simulink subsystem "ForwardDynamics"  (R2022a)
settings: Solver=VariableStepAuto  StartTime=0.0  StopTime=10.0  RelTol=1e-3
model mask{spaceRobot=SpaceRobot, SimulateUsing=Code generation}
  mask prompts: SimulateUsing "SystemBlock:MATLABSystem:SimulateUsing"
settings Model: Creator=charl  LastModifiedBy=charl

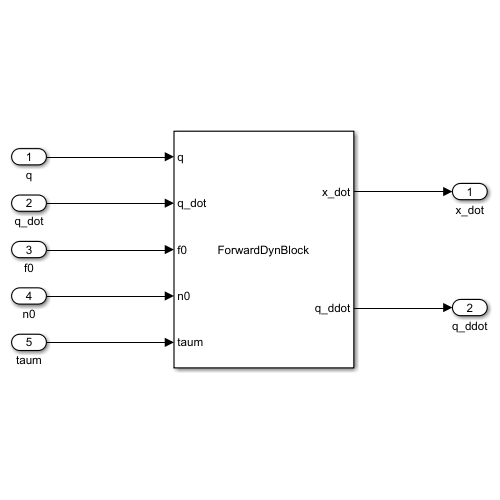
[thumbnail: Simulink's stored preview of the top-level diagram]
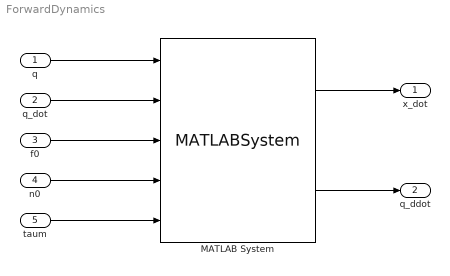
== system ForwardDynamics ==
  q : Inport
  q_dot : Inport  Port=2
  f0 : Inport  Port=3
  n0 : Inport  Port=4
  taum : Inport  Port=5
  MATLAB System : MATLABSystem  System=ForwardDynBlock  srInfo=srInfo  srInfoFunc=srInfoFunc  srStateFunc=srStateFunc  srStateFuncMex=srStateFuncMex  SimulateUsing=Code generation
      mask Type: ForwardDynBlock
      mask Display:
      | disp('ForwardDynBlock');
      | port_label('input',1,'q');
      | port_label('input',2,'q_dot');
      | port_label('input',3,'f0');
      | port_label('input',4,'n0');
      | port_label('input',5,'taum');
      | port_label('output',1,'x_dot');
      | port_label('output',2,'q_ddot');
  x_dot : Outport
  q_ddot : Outport  Port=2
  wires:
  f0/1 -> MATLAB System/3
  MATLAB System/1 -> x_dot/1
  n0/1 -> MATLAB System/4
  taum/1 -> MATLAB System/5
  q/1 -> MATLAB System/1
  q_dot/1 -> MATLAB System/2
  MATLAB System/2 -> q_ddot/1
